simulink model "variableStiffnessSystem"  (R2018a)
settings: Solver=VariableStepAuto  StartTime=0.0  StopTime=30  FixedStep=0.1  RelTol=1e-3
undefined symbols (not defined in the file or in its folder): J, Km, Kv, L, R
libraries: simulink x1
settings Model: Creator=pei-T  LastModifiedBy=pei-T

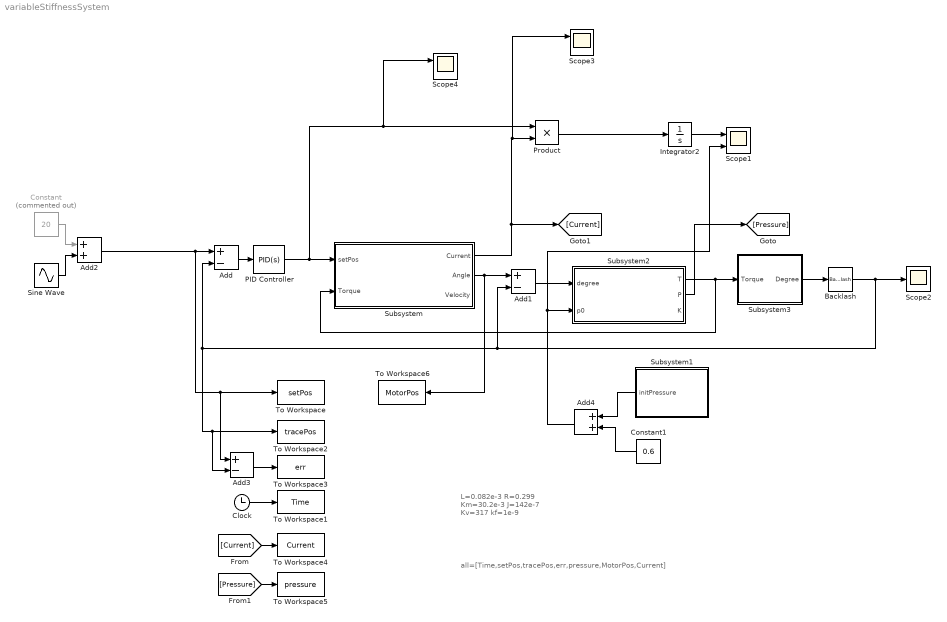
== system variableStiffnessSystem ==
  note: all=[Time,setPos,tracePos,err,pressure,MotorPos,Current]
  note: L=0.082e-3
      | R=0.299
      | Km=30.2e-3
      | J=142e-7
      | Kv=317
      | kf=1e-9
  Add : Sum  Inputs=+-
  Add1 : Sum  Inputs=+-
  Add2 : Sum
  Add3 : Sum  Inputs=+-
  Add4 : Sum
  Backlash : Backlash  BacklashWidth=4
  Clock : Clock
  Constant : Constant  Commented=on  Value=20
  Constant1 : Constant  Value=0.6
  Integrator2 : Integrator
  PID Controller : simulink/Continuous/PID Controller  Controller=PID  TimeDomain=Continuous-time  SampleTime=-1  IntegratorMethod=Forward Euler  FilterMethod=Forward Euler  Form=Parallel  UseFilter=on  ControllerParametersSource=internal  P=0.0356426855520821  I=0.176166294867686  D=0.00141630971712268  N=76.0880532204864  InitialConditionSource=internal  InitialConditionForIntegrator=0  InitialConditionForFilter=0  ExternalReset=none  LimitOutput=on  UpperSaturationLimit=24  LowerSaturationLimit=-24  LinearizeAsGain=on  AntiWindupMode=none  Kb=1  TrackingMode=off  Kt=1  PParamMin=[]  PParamMax=[]  IParamMin=[]  IParamMax=[]  DParamMin=[]  DParamMax=[]  NParamMin=[]  NParamMax=[]  KbParamMin=[]  KbParamMax=[]  KtParamMin=[]  KtParamMax=[]  POutMin=[]  POutMax=[]  IOutMin=[]  IOutMax=[]  DOutMin=[]  DOutMax=[]  NOutMin=[]  NOutMax=[]  KbOutMin=[]  KbOutMax=[]  KtOutMin=[]  KtOutMax=[]  IntegratorOutMin=[]  IntegratorOutMax=[]  FilterOutMin=[]  FilterOutMax=[]  SumOutMin=[]  SumOutMax=[]  SumI1OutMin=[]  SumI1OutMax=[]  SumI2OutMin=[]  SumI2OutMax=[]  SumI3OutMin=[]  SumI3OutMax=[]  SumDOutMin=[]  SumDOutMax=[]  SaturationOutMin=[]  SaturationOutMax=[]  IntegratorContinuousStateAttributes=''  IntegratorStateMustResolveToSignalObject=off  IntegratorRTWStateStorageClass=Auto  FilterContinuousStateAttributes=''  FilterStateMustResolveToSignalObject=off  FilterRTWStateStorageClass=Auto  DifferentiatorICPrevScaledInput=0  DifferentiatorOutMin=[]  DifferentiatorOutMax=[]  FilterDiffOutCoefMin=[]  FilterDiffOutCoefMax=[]  SumDenOutMin=[]  SumDenOutMax=[]  SumNumOutMin=[]  SumNumOutMax=[]  ReciprocalOutMin=[]  ReciprocalOutMax=[]  DivideOutMin=[]  DivideOutMax=[]  TunerSelectOption=Transfer Function Based (PID Tuner App)
  Product : Product
  Scope1 : Scope  NumInputPorts=2
  Scope2 : Scope
  Scope3 : Scope  NumInputPorts=2
  Scope4 : Scope  NumInputPorts=2
  Sine Wave : Sin  Amplitude=40  Frequency=0.5*pi  SampleTime=0
  Subsystem : Subsystem
  Subsystem1 : Subsystem
  Subsystem2 : Subsystem
  Subsystem3 : Subsystem
  To Workspace : ToWorkspace  VariableName=setPos  SampleTime=-1
      settings: Save2DSignal=2-D array (concatenate along first dimension)
  To Workspace1 : ToWorkspace  VariableName=Time  SampleTime=-1
      settings: Save2DSignal=2-D array (concatenate along first dimension)
  To Workspace2 : ToWorkspace  VariableName=tracePos  SampleTime=-1
      settings: Save2DSignal=2-D array (concatenate along first dimension)
  To Workspace3 : ToWorkspace  VariableName=err  SampleTime=-1
      settings: Save2DSignal=2-D array (concatenate along first dimension)
  To Workspace4 : ToWorkspace  VariableName=Current  SampleTime=-1
      settings: Save2DSignal=2-D array (concatenate along first dimension)
  To Workspace5 : ToWorkspace  VariableName=pressure  SampleTime=-1
      settings: Save2DSignal=2-D array (concatenate along first dimension)
  To Workspace6 : ToWorkspace  VariableName=MotorPos  SampleTime=-1
      settings: Save2DSignal=2-D array (concatenate along first dimension)
  wires:
  Subsystem2/1(T) -> Subsystem/2(Torque), Subsystem3/1(Torque)
  PID Controller/1 -> Scope4/1, Product/1, Subsystem/1(setPos)
  Add/1 -> PID Controller/1
  Subsystem/1(Current) -> Scope3/1, Product/2, [Current]
  Subsystem3/1(Degree) -> Backlash/1
  Add1/1 -> Subsystem2/1(degree)
  Constant/1 -> Add2/1
  Sine Wave/1 -> Add2/2
  Clock/1 -> To Workspace1/1
  [Pressure] -> To Workspace5/1
  [Current] -> To Workspace4/1
  Add3/1 -> To Workspace3/1
  Subsystem/2(Angle) -> To Workspace6/1, Add1/1
  Subsystem2/2(P) -> [Pressure]
  Add4/1 -> Scope1/2, Subsystem2/2(p0)
  Backlash/1 -> Add3/2, To Workspace2/1, Add/2, Add1/2, Scope2/1
  Product/1 -> Integrator2/1
  Integrator2/1 -> Scope1/1
  Add2/1 -> Add3/1, To Workspace/1, Add/1
  Constant1/1 -> Add4/2
  Subsystem1/1(initPressure) -> Add4/1

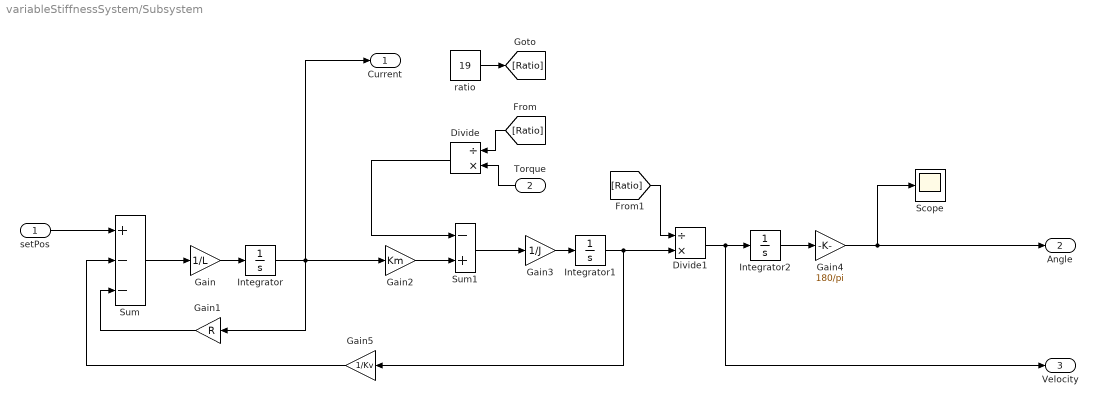
== system variableStiffnessSystem/Subsystem ==
  setPos : Inport
  Torque : Inport  Port=2
  Divide : Product  Inputs=/*
  Divide1 : Product  Inputs=/*
  Gain : Gain  Gain=1/L
  Gain1 : Gain  Gain=R
  Gain2 : Gain  Gain=Km
  Gain3 : Gain  Gain=1/J
  Gain4 : Gain  Gain=180/pi
  Gain5 : Gain  Gain=1/Kv
  Integrator : Integrator  LimitOutput=on  UpperSaturationLimit=80.2  LowerSaturationLimit=-80.2
  Integrator1 : Integrator
  Integrator2 : Integrator
  Scope : Scope
  Sum : Sum  Inputs=+--
  Sum1 : Sum  Inputs=-+
  ratio : Constant  Value=19
  Current : Outport
  Angle : Outport  Port=2
  Velocity : Outport  Port=3
  wires:
  Integrator2/1 -> Gain4/1
  setPos/1 -> Sum/1
  Divide1/1 -> Velocity/1, Integrator2/1
  Gain4/1 -> Angle/1, Scope/1
  Divide/1 -> Sum1/1
  [Ratio] -> Divide1/1
  Gain5/1 -> Sum/2
  Torque/1 -> Divide/2
  Gain2/1 -> Sum1/2
  Integrator/1 -> Current/1, Gain1/1, Gain2/1
  Integrator1/1 -> Divide1/2, Gain5/1
  Gain/1 -> Integrator/1
  Sum1/1 -> Gain3/1
  [Ratio] -> Divide/1
  Gain1/1 -> Sum/3
  Gain3/1 -> Integrator1/1
  Sum/1 -> Gain/1
  ratio/1 -> [Ratio]

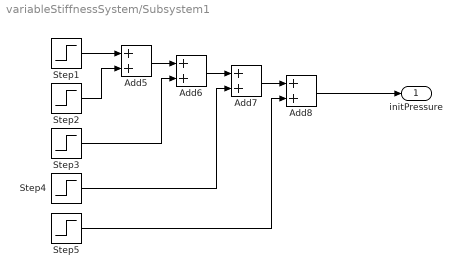
== system variableStiffnessSystem/Subsystem1 ==
  Add{5..8} (4 alike) : Sum
  Step1 : Step  Time=5  After=0.1  SampleTime=0
  Step2 : Step  Time=10  After=0.1  SampleTime=0
  Step3 : Step  Time=15  After=0.1  SampleTime=0
  Step4 : Step  Time=20  After=0.1  SampleTime=0
  Step5 : Step  Time=25  After=0.1  SampleTime=0
  initPressure : Outport
  wires:
  Add7/1 -> Add8/1
  Step2/1 -> Add5/2
  Add6/1 -> Add7/1
  Step3/1 -> Add6/2
  Add5/1 -> Add6/1
  Step4/1 -> Add7/2
  Step1/1 -> Add5/1
  Step5/1 -> Add8/2
  Add8/1 -> initPressure/1

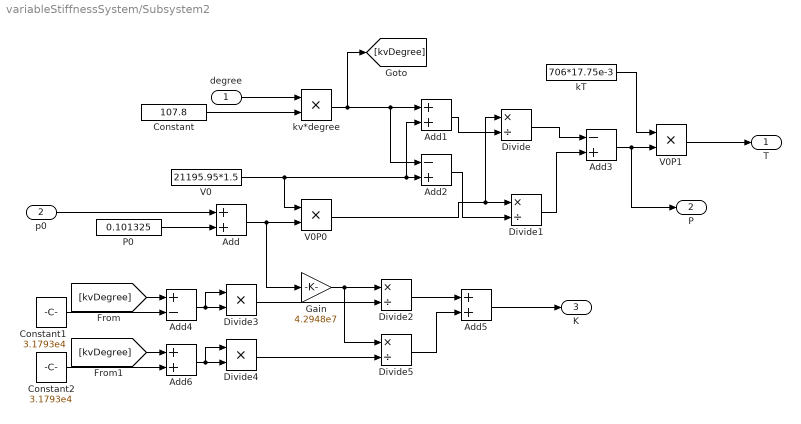
== system variableStiffnessSystem/Subsystem2 ==
  degree : Inport
  p0 : Inport  Port=2
  Add{,1,5..6} (4 alike) : Sum
  Add2 : Sum  Inputs=-+
  Add3 : Sum  Inputs=-+
  Add4 : Sum  Inputs=+-
  Constant : Constant  Value=107.8
  Constant1 : Constant  Value=3.1793e4
  Constant2 : Constant  Value=3.1793e4
  Divide{,1..2,5} (4 alike) : Product  Inputs=*/
  Divide3 : Product  Inputs=**
  Divide4 : Product  Inputs=**
  Gain : Gain  Gain=4.2948e7
  P0 : Constant  Value=0.101325
  V0 : Constant  Value=21195.95*1.5
  V0P0 : Product
  V0P1 : Product
  kT : Constant  Value=706*17.75e-3
  kv*degree : Product
  T : Outport
  P : Outport  Port=2
  K : Outport  Port=3
  wires:
  Add3/1 -> P/1, V0P1/2
  V0/1 -> V0P0/1, Add2/2, Add1/2
  V0P1/1 -> T/1
  p0/1 -> Add/1
  Constant/1 -> kv*degree/2
  degree/1 -> kv*degree/1
  Add/1 -> Gain/1, V0P0/2
  P0/1 -> Add/2
  kv*degree/1 -> [kvDegree], Add2/1, Add1/1
  kT/1 -> V0P1/1
  V0P0/1 -> Divide1/1, Divide/1
  Add2/1 -> Divide1/2
  Add1/1 -> Divide/2
  Divide1/1 -> Add3/2
  Divide/1 -> Add3/1
  Gain/1 -> Divide5/1, Divide2/1
  [kvDegree] -> Add4/1
  Constant1/1 -> Add4/2
  Add4/1 -> Divide3/1, Divide3/2
  Divide3/1 -> Divide2/2
  Divide2/1 -> Add5/1
  Add6/1 -> Divide4/1, Divide4/2
  [kvDegree] -> Add6/1
  Constant2/1 -> Add6/2
  Divide4/1 -> Divide5/2
  Divide5/1 -> Add5/2
  Add5/1 -> K/1

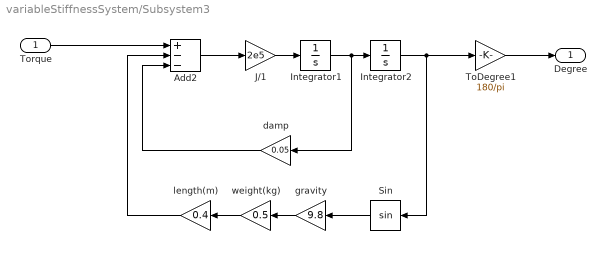
== system variableStiffnessSystem/Subsystem3 ==
  Torque : Inport
  Add2 : Sum  Inputs=+--
  Integrator1 : Integrator
  Integrator2 : Integrator
  J/1 : Gain  Gain=2e5
  Sin : Trigonometry
  ToDegree1 : Gain  Gain=180/pi
  damp : Gain  Gain=0.05
  gravity : Gain  Gain=9.8
  length(m) : Gain  Gain=0.4
  weight(kg) : Gain  Gain=0.5
  Degree : Outport
  wires:
  J/1/1 -> Integrator1/1
  Add2/1 -> J/1/1
  Torque/1 -> Add2/1
  damp/1 -> Add2/3
  Sin/1 -> gravity/1
  Integrator1/1 -> damp/1, Integrator2/1
  weight(kg)/1 -> length(m)/1
  length(m)/1 -> Add2/2
  Integrator2/1 -> Sin/1, ToDegree1/1
  gravity/1 -> weight(kg)/1
  ToDegree1/1 -> Degree/1
